simulink library "TrebleBoost"  (R2022b)
settings: Solver=VariableStepAuto  StartTime=0.0  StopTime=10.0  RelTol=1e-3
undefined symbols (not defined in the file or in its folder): magnitude, Row, TrebleBoost51Config, TrebleBoostConfig
libraries: TuneVar x30, TOP x12, StateVar x4, HandyTextFile x2, FeaturePath x2, PooliirLib x2, $bdroot x1, dspmtrx3 x1, dspxfrm3 x1
settings Model: Creator=jk1043656  LastModifiedBy=sc48041
settings SolverCC: AlgebraicLoopSolver=TrustRegion
settings DataIOCC: ReturnWorkspaceOutputs=off
settings DebuggingCC: UnconnectedInputMsg=warning  UnconnectedOutputMsg=warning  UnconnectedLineMsg=warning  SFMachineParentedDataDiag=warning  ArithmeticOperatorsInVariantConditions=warning
settings ModelReferenceCC: EnableRefExpFcnMdlSchedulingChecks=on
settings SFSimCC: CustomCodeUndefinedFunction=UseInterfaceOnly

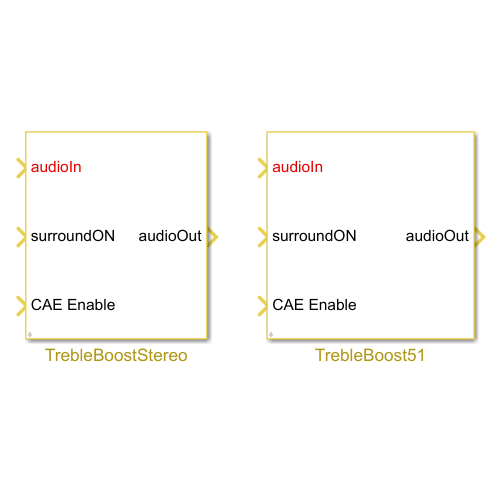
[thumbnail: Simulink's stored preview of the top-level diagram]
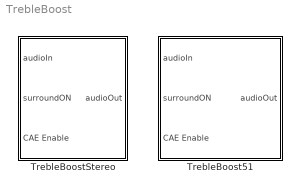
== system TrebleBoost ==
  TrebleBoost51 : Subsystem  mask{Config=TrebleBoost51Config}
      mask prompts: Config "TrebleBoost51Config"
      mask init:
      | blkh=gcbh;
      | Config=BTConfig.Assert(blkh,Config);
      | 
      | Config.Validate();
  TrebleBoostStereo : Subsystem  mask{Config=TrebleBoostConfig}
      mask prompts: Config "TrebleBoostStereoConfig"
      mask init:
      | blkh=gcbh;
      | Config=BTConfig.Assert(blkh,Config);
      | 
      | Config.Validate();

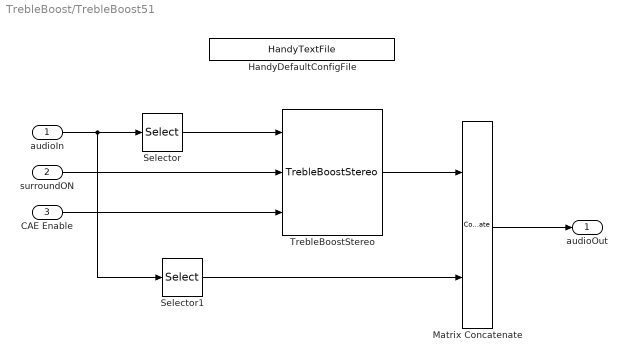
== system TrebleBoost/TrebleBoost51 ==
  audioIn : Inport  OutDataTypeStr=single
  surroundON : Inport  Port=2
  CAE Enable : Inport  Port=3
  HandyDefaultConfigFile : HandyTextFile/HandyTextFile  TemplateSource=Config  FileSuffix=Init  OpenDialogOnLoad=off  UseThisBlockName=off  AddGrandParentNamePrefix=off  TheDefaultText=|  ShowInLibBrowser=on
      | % $(FILENAME) Setup model parameters for each "Init" callback (e.g. update diagram)
      | sample_rate_in_hertz = 44100;
      | frame_size = 32;
      | sysin_channel_count = 2;
      settings: SourceProductName=Bose Talaria
  Matrix Concatenate : Concatenate  Mode=Multidimensional array  ConcatenateDimension=2
  Selector : Selector  NumberOfDimensions=2  InputPortWidth=3  IndexOptions=Select all,Index vector (dialog)  Indices=[1 3],[1 2]  OutputSizes=1,1
  Selector1 : Selector  NumberOfDimensions=2  InputPortWidth=3  IndexOptions=Select all,Index vector (dialog)  Indices=[1 3],3:6  OutputSizes=1,1
  TrebleBoostStereo : $bdroot/TrebleBoostStereo  Config=Config
  audioOut : Outport  OutDataTypeStr=single  VectorParamsAs1DForOutWhenUnconnected=off
  wires:
  Matrix Concatenate/1 -> audioOut/1
  Selector1/1 -> Matrix Concatenate/2
  audioIn/1 -> Selector/1, Selector1/1
  TrebleBoostStereo/1 -> Matrix Concatenate/1
  Selector/1 -> TrebleBoostStereo/1
  surroundON/1 -> TrebleBoostStereo/2
  CAE Enable/1 -> TrebleBoostStereo/3

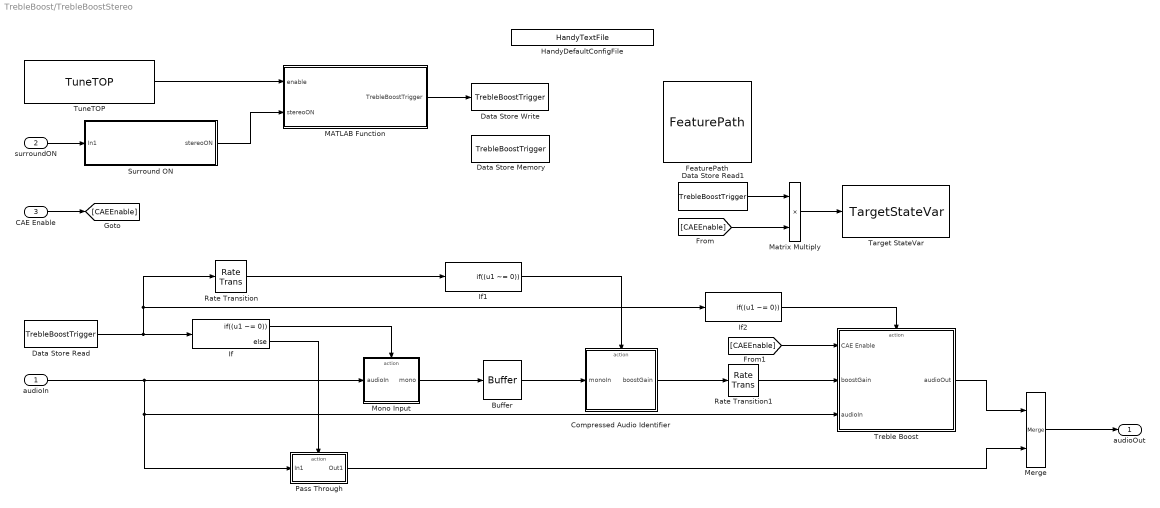
== system TrebleBoost/TrebleBoostStereo ==
  audioIn : Inport  OutDataTypeStr=single  PortDimensions=[32 2]
  surroundON : Inport  Port=2
  CAE Enable : Inport  Port=3
  Buffer : Buffer  N=Config.FftFrameSize  OutputFrames=off
  Compressed Audio Identifier : Subsystem  TreatAsAtomicUnit=on
  Data Store Memory : DataStoreMemory  DataStoreName=TrebleBoostTrigger  ReadBeforeWriteMsg=warning  WriteAfterWriteMsg=warning  WriteAfterReadMsg=warning  InitialValue=1  ShowAdditionalParam=off
  Data Store Read : DataStoreRead  DataStoreName=TrebleBoostTrigger  IndexOptions=Index vector (dialog)  Indices=1  OutputSizes=1
  Data Store Read1 : DataStoreRead  DataStoreName=TrebleBoostTrigger  IndexOptions=Index vector (dialog)  Indices=1  OutputSizes=1
  Data Store Write : DataStoreWrite  DataStoreName=TrebleBoostTrigger  IndexOptions=Index vector (dialog)  Indices=1  OutputSizes=1
  FeaturePath : FeaturePath/FeaturePath  FeatureName=TrebleBoost  IsGroup=off  GroupNumber=-1  IsModule=off  TriggerInit=[2025 269 2140 376]
      settings: SourceProductName=Bose Talaria
  HandyDefaultConfigFile : HandyTextFile/HandyTextFile  TemplateSource=Config  FileSuffix=Init  OpenDialogOnLoad=off  UseThisBlockName=off  AddGrandParentNamePrefix=off  TheDefaultText=|  ShowInLibBrowser=on
      | % $(FILENAME) Setup model parameters for each "Init" callback (e.g. update diagram)
      | sample_rate_in_hertz = 44100;
      | frame_size = 32;
      | sysin_channel_count = 2;
      settings: SourceProductName=Bose Talaria
  If : If  IfExpression=(u1 ~= 0)
  If1 : If  IfExpression=(u1 ~= 0)  ShowElse=off
  If2 : If  IfExpression=(u1 ~= 0)  ShowElse=off
  MATLAB Function : MATLAB Function  TreatAsAtomicUnit=on
  Matrix Multiply : Product  OutDataTypeStr=double
  Merge : Merge
  Mono Input : Subsystem  TreatAsAtomicUnit=on
  Pass Through : Subsystem  TreatAsAtomicUnit=on
  Rate Transition : RateTransition  Integrity=off  OutPortSampleTimeOpt=Multiple of input port sample time  OutPortSampleTimeMultiple=8
  Rate Transition1 : RateTransition  Integrity=off  OutPortSampleTimeOpt=Multiple of input port sample time  OutPortSampleTimeMultiple=1/8
  Surround ON : Subsystem
  Target StateVar : StateVar/TargetStateVar  TriggerInit=[2260 406 2400 474]  TspName=Enable  StateName=Enable  UseSameName=on  IfdefMacro=[]
      settings: SourceProductName=Bose Talaria
  Treble Boost : Subsystem  TreatAsAtomicUnit=on
  TuneTOP : TuneVar/TuneTOP  TriggerInit=[1190 242 1360 298]  TopName=EnableFlag  TuneName=EnableFlag  DataTypeOut=int32  TunabilityNumber=1  MinValue=[]  MaxValue=[]  BankNumber=0  PreOverlay=false  PostOverlay=false  UseSameName=on  MaskValue=Config.DefaultTuning.EnableFlag
      settings: SourceProductName=Bose Talaria
  audioOut : Outport  OutDataTypeStr=single  VectorParamsAs1DForOutWhenUnconnected=off
  wires:
  Rate Transition/1 -> If1/1
  If/2 -> Pass Through/Action
  MATLAB Function/1(TrebleBoostTrigger) -> Data Store Write/1
  Merge/1 -> audioOut/1
  Data Store Read/1 -> If/1, If2/1, Rate Transition/1
  Pass Through/1(Out1) -> Merge/2
  If2/1 -> Treble Boost/Action
  Treble Boost/1(audioOut) -> Merge/1
  Compressed Audio Identifier/1(boostGain) -> Rate Transition1/1
  Buffer/1 -> Compressed Audio Identifier/1(monoIn)
  Mono Input/1(mono) -> Buffer/1
  Rate Transition1/1 -> Treble Boost/2(boostGain)
  Surround ON/1(stereoON) -> MATLAB Function/2(stereoON)
  If/1 -> Mono Input/Action
  If1/1 -> Compressed Audio Identifier/Action
  surroundON/1 -> Surround ON/1(In1)
  audioIn/1 -> Pass Through/1(In1), Treble Boost/3(audioIn), Mono Input/1(audioIn)
  TuneTOP/1 -> MATLAB Function/1(enable)
  CAE Enable/1 -> [CAEEnable]
  [CAEEnable] -> Treble Boost/1(CAE Enable)
  Data Store Read1/1 -> Matrix Multiply/1
  [CAEEnable] -> Matrix Multiply/2
  Matrix Multiply/1 -> Target StateVar/1

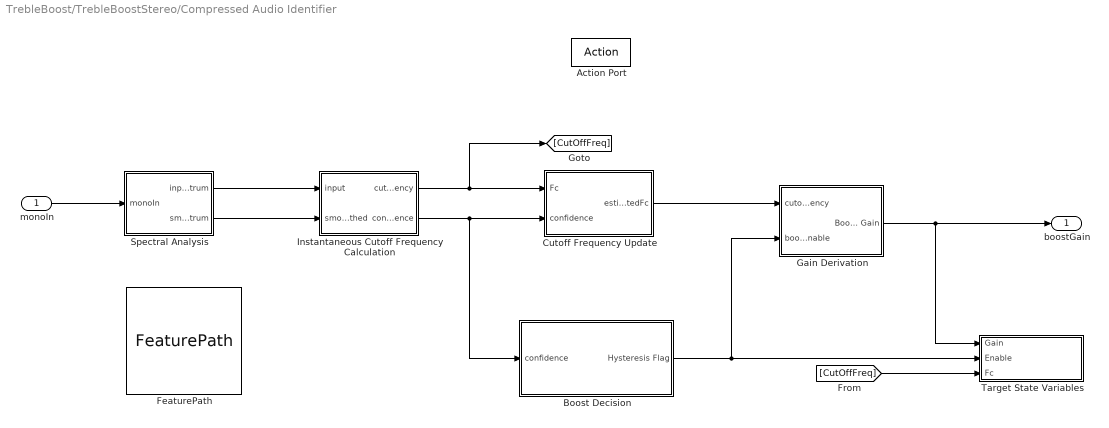
== system TrebleBoost/TrebleBoostStereo/Compressed Audio Identifier ==
  monoIn : Inport
  Action Port : ActionPort
  Boost Decision : Subsystem
  Cutoff Frequency Update : Subsystem
  FeaturePath : FeaturePath/FeaturePath  FeatureName=Identifier  IsGroup=off  GroupNumber=-1  IsModule=off  TriggerInit=[-155 264 -40 371]
      settings: SourceProductName=Bose Talaria
  Gain Derivation : Subsystem
  Instantaneous Cutoff Frequency Calculation : Subsystem
  Spectral Analysis : Subsystem
  Target State Variables : Subsystem
  boostGain : Outport  VectorParamsAs1DForOutWhenUnconnected=off
  wires:
  Gain Derivation/1(Boost Gain) -> boostGain/1, Target State Variables/1(Gain)
  Boost Decision/1(Hysteresis Flag) -> Gain Derivation/2(boostEnable), Target State Variables/2(Enable)
  Cutoff Frequency Update/1(estimatedFc) -> Gain Derivation/1(cutoffFrequency)
  Instantaneous Cutoff Frequency Calculation/1(cutoffFrequency) -> [CutOffFreq], Cutoff Frequency Update/1(Fc)
  monoIn/1 -> Spectral Analysis/1(monoIn)
  Instantaneous Cutoff Frequency Calculation/2(confidence) -> Boost Decision/1(confidence), Cutoff Frequency Update/2(confidence)
  Spectral Analysis/1(inputSpectrum) -> Instantaneous Cutoff Frequency Calculation/1(input)
  Spectral Analysis/2(smoothedSpectrum) -> Instantaneous Cutoff Frequency Calculation/2(smoothed)
  [CutOffFreq] -> Target State Variables/3(Fc)

== system TrebleBoost/TrebleBoostStereo/Mono Input ==
  audioIn : Inport
  Action Port : ActionPort
  Sum of Elements : Sum  Inputs=+  CollapseMode=Specified dimension  CollapseDim=2
  mono : Outport  VectorParamsAs1DForOutWhenUnconnected=off
  wires:
  audioIn/1 -> Sum of Elements/1
  Sum of Elements/1 -> mono/1

== system TrebleBoost/TrebleBoostStereo/Pass Through ==
  In1 : Inport
  Action Port : ActionPort
  Out1 : Outport  VectorParamsAs1DForOutWhenUnconnected=off
  wires:
  In1/1 -> Out1/1

== system TrebleBoost/TrebleBoostStereo/Surround ON ==
  In1 : Inport
  TOP : TOP/TOP  TriggerInit=[440 20 585 80]  TopName=StereoON  DataType=int32  BankNumber=0  PreOverlay=false  PostOverlay=false  Role=Automatic
      settings: SourceProductName=Bose Talaria
  TranslateTrigger : TuneVar/TranslateTrigger  TriggerInit=[306 -100 344 -45]
      settings: SourceProductName=Bose Talaria
  Trivial Translation : MATLAB Function  TreatAsAtomicUnit=on
  stereoON : Outport  VectorParamsAs1DForOutWhenUnconnected=off
  wires:
  TranslateTrigger/1 -> Trivial Translation/Trigger
  Trivial Translation/1(isStereo) -> TOP/1
  In1/1 -> Trivial Translation/1(surroundOn)  "SurroundON"
  TOP/1 -> stereoON/1  "StereoON"

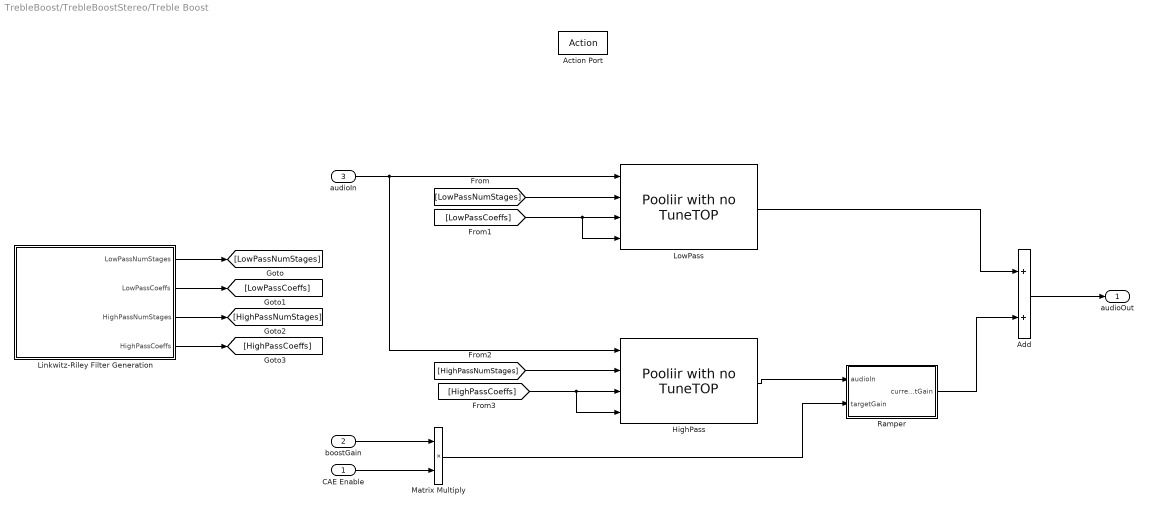
== system TrebleBoost/TrebleBoostStereo/Treble Boost ==
  CAE Enable : Inport
  boostGain : Inport  Port=2
  audioIn : Inport  Port=3
  Action Port : ActionPort
  Add : Sum
  HighPass : PooliirLib/Pooliir with no TuneTOP  maxNumStages=Config.MaxNumStages  variantType=Config.Variant
  Linkwitz-Riley Filter Generation : Subsystem
  LowPass : PooliirLib/Pooliir with no TuneTOP  maxNumStages=Config.MaxNumStages  variantType=Config.Variant
  Matrix Multiply : Product
  Ramper : Subsystem
  audioOut : Outport  VectorParamsAs1DForOutWhenUnconnected=off
  wires:
  Ramper/1(currentGain) -> Add/2
  HighPass/1 -> Ramper/1(audioIn)
  Linkwitz-Riley Filter Generation/3(HighPassNumStages) -> [HighPassNumStages]
  Linkwitz-Riley Filter Generation/1(LowPassNumStages) -> [LowPassNumStages]
  audioIn/1 -> LowPass/1, HighPass/1
  LowPass/1 -> Add/1
  [LowPassNumStages] -> LowPass/2
  [HighPassCoeffs] -> HighPass/4, HighPass/3
  Linkwitz-Riley Filter Generation/4(HighPassCoeffs) -> [HighPassCoeffs]
  [HighPassNumStages] -> HighPass/2
  Linkwitz-Riley Filter Generation/2(LowPassCoeffs) -> [LowPassCoeffs]
  [LowPassCoeffs] -> LowPass/4, LowPass/3
  Add/1 -> audioOut/1
  CAE Enable/1 -> Matrix Multiply/2
  boostGain/1 -> Matrix Multiply/1
  Matrix Multiply/1 -> Ramper/2(targetGain)

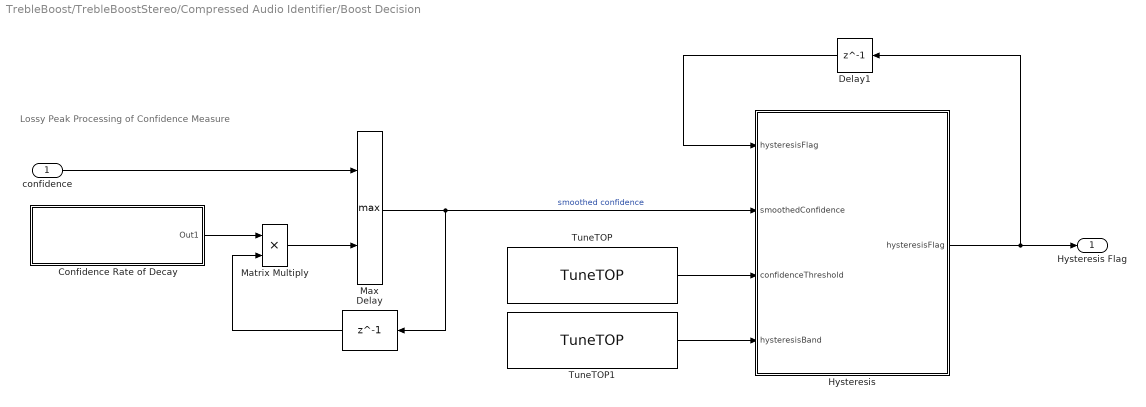
== system TrebleBoost/TrebleBoostStereo/Compressed Audio Identifier/Boost Decision ==
  note: Lossy Peak Processing of Confidence Measure
  confidence : Inport
  Confidence Rate of Decay : Subsystem
  Delay : Delay  DelayLength=1  InitialCondition=0
  Delay1 : Delay  DelayLength=1  InitialCondition=1
  Hysteresis : MATLAB Function  TreatAsAtomicUnit=on
  Matrix Multiply : Product
  Max : MinMax  Function=max  Inputs=2
  TuneTOP : TuneVar/TuneTOP  TriggerInit=[355 142 525 198]  TopName=ConfidenceThreshold  TuneName=ConfidenceThreshold  DataType=single  TunabilityNumber=1  MinValue=[]  MaxValue=[]  BankNumber=0  PreOverlay=false  PostOverlay=false  UseSameName=on  MaskValue=Config.DefaultTuning.ConfidenceThreshold
      settings: SourceProductName=Bose Talaria
  TuneTOP1 : TuneVar/TuneTOP  TriggerInit=[355 207 525 263]  TopName=HysteresisBand  TuneName=HysteresisBand  DataType=single  TunabilityNumber=1  MinValue=[]  MaxValue=[]  BankNumber=0  PreOverlay=false  PostOverlay=false  UseSameName=on  MaskValue=Config.DefaultTuning.HysteresisBand
      settings: SourceProductName=Bose Talaria
  Hysteresis Flag : Outport  VectorParamsAs1DForOutWhenUnconnected=off
  wires:
  Hysteresis/1(hysteresisFlag) -> Hysteresis Flag/1, Delay1/1
  TuneTOP1/1 -> Hysteresis/4(hysteresisBand)
  Matrix Multiply/1 -> Max/2
  Max/1 -> Delay/1, Hysteresis/2(smoothedConfidence)  "smoothed confidence"
  Confidence Rate of Decay/1(Out1) -> Matrix Multiply/1
  Delay/1 -> Matrix Multiply/2
  confidence/1 -> Max/1
  TuneTOP/1 -> Hysteresis/3(confidenceThreshold)
  Delay1/1 -> Hysteresis/1("hysteresisFlag ")

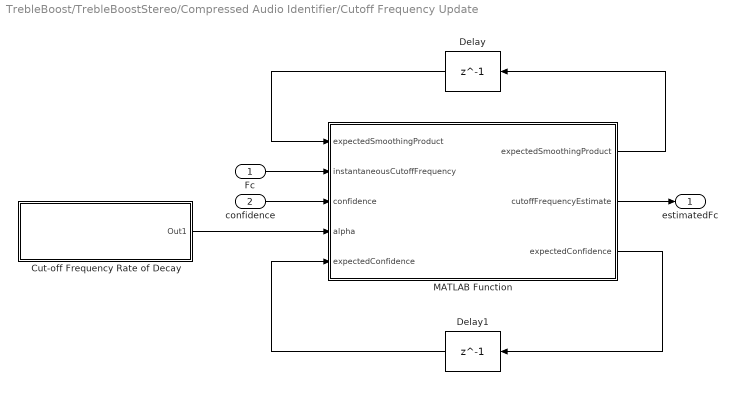
== system TrebleBoost/TrebleBoostStereo/Compressed Audio Identifier/Cutoff Frequency Update ==
  Fc : Inport
  confidence : Inport  Port=2
  Cut-off Frequency Rate of Decay : Subsystem
  Delay : Delay  DelayLength=1  InitialCondition=0
  Delay1 : Delay  DelayLength=1  InitialCondition=0
  MATLAB Function : MATLAB Function  TreatAsAtomicUnit=on
  estimatedFc : Outport  VectorParamsAs1DForOutWhenUnconnected=off
  wires:
  Cut-off Frequency Rate of Decay/1(Out1) -> MATLAB Function/4(alpha)
  confidence/1 -> MATLAB Function/3(confidence)
  Fc/1 -> MATLAB Function/2(instantaneousCutoffFrequency)
  MATLAB Function/3(expectedConfidence) -> Delay1/1
  Delay1/1 -> MATLAB Function/5("expectedConfidence ")
  Delay/1 -> MATLAB Function/1("expectedSmoothingProduct ")
  MATLAB Function/2(cutoffFrequencyEstimate) -> estimatedFc/1
  MATLAB Function/1(expectedSmoothingProduct) -> Delay/1

== system TrebleBoost/TrebleBoostStereo/Compressed Audio Identifier/Gain Derivation ==
  cutoffFrequency : Inport
  boostEnable : Inport  Port=2
  MATLAB Function : MATLAB Function  TreatAsAtomicUnit=on
  Subsystem : Subsystem
  Boost Gain : Outport  VectorParamsAs1DForOutWhenUnconnected=off
  wires:
  boostEnable/1 -> MATLAB Function/1(boostEnable)
  MATLAB Function/1(boostGain) -> Boost Gain/1
  Subsystem/1(Freq1InHz) -> MATLAB Function/3(Freq1Hz)
  Subsystem/2(Freq2InHz) -> MATLAB Function/4(Freq2Hz)
  Subsystem/3(Freq3InHz) -> MATLAB Function/5(Freq3Hz)
  Subsystem/4(Gain1IndB) -> MATLAB Function/6(Gain1dB)
  Subsystem/5(Gain2IndB) -> MATLAB Function/7(Gain2dB)
  cutoffFrequency/1 -> MATLAB Function/2(cutoffFrequency)

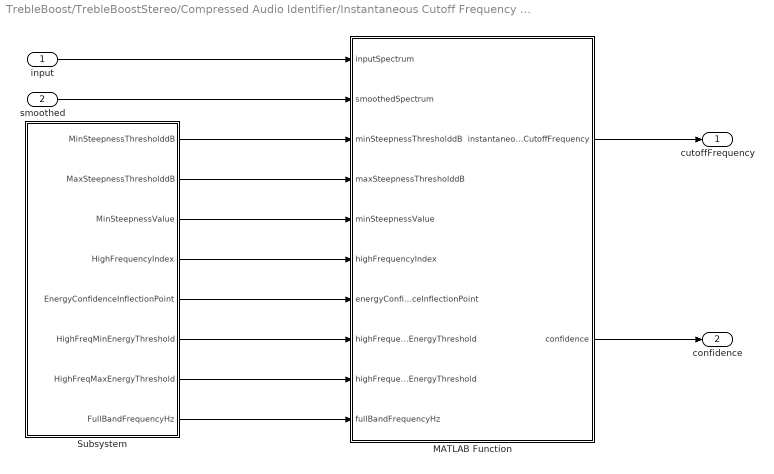
== system TrebleBoost/TrebleBoostStereo/Compressed Audio Identifier/Instantaneous Cutoff Frequency Calculation ==
  input : Inport
  smoothed : Inport  Port=2
  MATLAB Function : MATLAB Function  TreatAsAtomicUnit=on  mask{minDetectionFrequencyIndex=Config.MinDetectionFrequencyIndex, maxDetectionFrequencyIndex=Config.MaxDetectionFrequencyIndex, spectrumSize=Config.SpectrumSize, frequencies=Config.Frequencies, steepnessIndexRange=Config.SteepnessIndexRange}
  Subsystem : Subsystem
  cutoffFrequency : Outport  VectorParamsAs1DForOutWhenUnconnected=off
  confidence : Outport  Port=2  OutDataTypeStr=single  VectorParamsAs1DForOutWhenUnconnected=off
  wires:
  input/1 -> MATLAB Function/1(inputSpectrum)
  Subsystem/4(HighFrequencyIndex) -> MATLAB Function/6(highFrequencyIndex)
  Subsystem/8(FullBandFrequencyHz) -> MATLAB Function/10(fullBandFrequencyHz)
  Subsystem/7(HighFreqMaxEnergyThreshold) -> MATLAB Function/9(highFrequencyMaxEnergyThreshold)
  Subsystem/6(HighFreqMinEnergyThreshold) -> MATLAB Function/8(highFrequencyMinEnergyThreshold)
  Subsystem/5(EnergyConfidenceInflectionPoint) -> MATLAB Function/7(energyConfidenceInflectionPoint)
  Subsystem/3(MinSteepnessValue) -> MATLAB Function/5(minSteepnessValue)
  Subsystem/1(MinSteepnessThresholddB) -> MATLAB Function/3(minSteepnessThresholddB)
  MATLAB Function/2(confidence) -> confidence/1
  Subsystem/2(MaxSteepnessThresholddB) -> MATLAB Function/4(maxSteepnessThresholddB)
  MATLAB Function/1(instantaneousCutoffFrequency) -> cutoffFrequency/1
  smoothed/1 -> MATLAB Function/2(smoothedSpectrum)

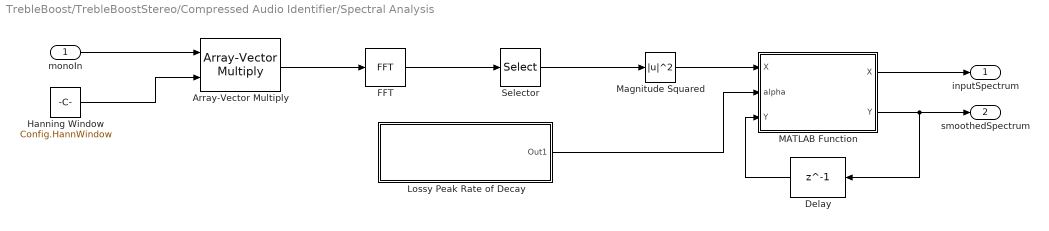
== system TrebleBoost/TrebleBoostStereo/Compressed Audio Identifier/Spectral Analysis ==
  monoIn : Inport
  Array-Vector Multiply : dspmtrx3/Array-Vector Multiply  mode=Mute  saveAsFlag=0  Dimension=1  V_Source=Input port  V_VectFromMask=[0.5 0.25]  roundingMode=Floor  overflowMode=off  firstCoeffSignedness=Auto  firstCoeffDataTypeStr=Inherit: Same word length as input  firstCoeffMin=[]  firstCoeffMax=[]  firstCoeffLastDataTypeStr=Inherit: Same word length as input  prodOutputSignedness=Auto  accumSignedness=Auto  outputSignedness=Auto  outputMin=[]  outputMax=[]
  Delay : Delay  DelayLength=1  InitialCondition=zeros(1, Config.SpectrumSize, 'single')
  FFT : dspxfrm3/FFT  FFTImplementation=Auto  CompMethod=Table lookup  TableOpt=NEW  TableOptActive=Speed  BitRevOrder=off  Normalize=off  InheritFFTLength=on  FFTLength=64  WrapInput=on  roundingMode=Floor  overflowMode=off  firstCoeffDataTypeStr=Inherit: Same word length as input  firstCoeffLastDataTypeStr=Inherit: Same word length as input  outputMin=[]  outputMax=[]
  Hanning Window : Constant  Value=Config.HannWindow  VectorParams1D=off  OutDataTypeStr=single  SampleTime=Inf
  Lossy Peak Rate of Decay : Subsystem
  MATLAB Function : MATLAB Function  TreatAsAtomicUnit=on  mask{spectrumSize=Config.SpectrumSize}
  Magnitude Squared : Math  Operator=magnitude^2  SignedPower=on
  Selector : Selector  NumberOfDimensions=2  InputPortWidth=3  IndexOptions=Index vector (dialog),Select all  Indices=1:Config.SpectrumSize,1  OutputSizes=1,1
  inputSpectrum : Outport  VectorParamsAs1DForOutWhenUnconnected=off
  smoothedSpectrum : Outport  Port=2  VectorParamsAs1DForOutWhenUnconnected=off
  wires:
  Array-Vector Multiply/1 -> FFT/1
  monoIn/1 -> Array-Vector Multiply/1
  FFT/1 -> Selector/1
  Hanning Window/1 -> Array-Vector Multiply/2
  Lossy Peak Rate of Decay/1(Out1) -> MATLAB Function/2(alpha)
  Magnitude Squared/1 -> MATLAB Function/1("X ")
  Selector/1 -> Magnitude Squared/1
  MATLAB Function/2(Y) -> smoothedSpectrum/1, Delay/1
  Delay/1 -> MATLAB Function/3("Y ")
  MATLAB Function/1(X) -> inputSpectrum/1

== system TrebleBoost/TrebleBoostStereo/Compressed Audio Identifier/Target State Variables ==
  Gain : Inport
  Enable : Inport  Port=2
  Fc : Inport  Port=3
  Target StateVar : StateVar/TargetStateVar  TriggerInit=[360 81 500 149]  TspName=BoostEnable  StateName=BoostEnable  UseSameName=on  IfdefMacro=[]
      settings: SourceProductName=Bose Talaria
  Target StateVar1 : StateVar/TargetStateVar  TriggerInit=[360 -4 500 64]  TspName=BoostGain  StateName=BoostGain  UseSameName=on  IfdefMacro=[]
      settings: SourceProductName=Bose Talaria
  Target StateVar2 : StateVar/TargetStateVar  TriggerInit=[360 166 500 234]  TspName=CutOffFrequency  StateName=CutOffFrequency  UseSameName=on  IfdefMacro=[]
      settings: SourceProductName=Bose Talaria
  wires:
  Fc/1 -> Target StateVar2/1
  Gain/1 -> Target StateVar1/1
  Enable/1 -> Target StateVar/1

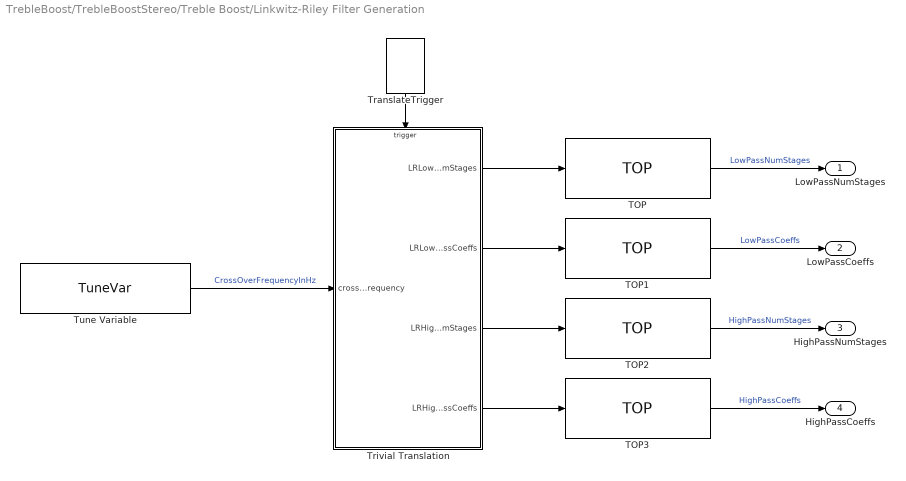
== system TrebleBoost/TrebleBoostStereo/Treble Boost/Linkwitz-Riley Filter Generation ==
  TOP : TOP/TOP  TriggerInit=[490 -25 635 35]  TopName=LowPassNumStages  DataType=uint32  BankNumber=0  PreOverlay=false  PostOverlay=false  Role=Automatic
      settings: SourceProductName=Bose Talaria
  TOP1 : TOP/TOP  TriggerInit=[490 55 635 115]  TopName=LowPassCoeffs  DataType=single  BankNumber=0  PreOverlay=false  PostOverlay=false  Role=Automatic
      settings: SourceProductName=Bose Talaria
  TOP2 : TOP/TOP  TriggerInit=[490 135 635 195]  TopName=HighPassNumStages  DataType=uint32  BankNumber=0  PreOverlay=false  PostOverlay=false  Role=Automatic
      settings: SourceProductName=Bose Talaria
  TOP3 : TOP/TOP  TriggerInit=[490 215 635 275]  TopName=HighPassCoeffs  DataType=single  BankNumber=0  PreOverlay=false  PostOverlay=false  Role=Automatic
      settings: SourceProductName=Bose Talaria
  TranslateTrigger : TuneVar/TranslateTrigger  TriggerInit=[311 -125 349 -70]
      settings: SourceProductName=Bose Talaria
  Trivial Translation : MATLAB Function  TreatAsAtomicUnit=on  mask{filterOrder=Config.FilterOrder, sampleRate=Config.SampleRate, maxNumStages=Config.MaxNumStages, numChannels=Config.NumChannels}
  Tune Variable : TuneVar/TuneVar  TuneName=CrossOverFrequencyInHz  SpecifyMaxSize=off  VariableDim=1 (Row)  MaxSize=[1 1]  TunabilityNumber=1  MinValue=[]  MaxValue=[]  TriggerInit=[-55 100 115 150]  MaskValue=Config.DefaultTuning.CrossOverFrequency
      settings: SourceProductName=Bose Talaria
  LowPassNumStages : Outport  VectorParamsAs1DForOutWhenUnconnected=off
  LowPassCoeffs : Outport  Port=2  VectorParamsAs1DForOutWhenUnconnected=off
  HighPassNumStages : Outport  Port=3  VectorParamsAs1DForOutWhenUnconnected=off
  HighPassCoeffs : Outport  Port=4  VectorParamsAs1DForOutWhenUnconnected=off
  wires:
  Trivial Translation/4(LRHighPassCoeffs) -> TOP3/1
  Trivial Translation/3(LRHighPassNumStages) -> TOP2/1
  Trivial Translation/2(LRLowPassCoeffs) -> TOP1/1
  TOP3/1 -> HighPassCoeffs/1  "HighPassCoeffs"
  TOP2/1 -> HighPassNumStages/1  "HighPassNumStages"
  TOP1/1 -> LowPassCoeffs/1  "LowPassCoeffs"
  TranslateTrigger/1 -> Trivial Translation/Trigger
  Trivial Translation/1(LRLowPassNumStages) -> TOP/1
  Tune Variable/1 -> Trivial Translation/1(crossOverFrequency)  "CrossOverFrequencyInHz"
  TOP/1 -> LowPassNumStages/1  "LowPassNumStages"

== system TrebleBoost/TrebleBoostStereo/Treble Boost/Ramper ==
  audioIn : Inport
  targetGain : Inport  Port=2
  MATLAB Function : MATLAB Function  TreatAsAtomicUnit=on
  Ramp Coefficient : Subsystem
  currentGain : Outport  VectorParamsAs1DForOutWhenUnconnected=off
  wires:
  MATLAB Function/1(audioOut) -> currentGain/1
  targetGain/1 -> MATLAB Function/2(targetGain)
  audioIn/1 -> MATLAB Function/1(audioIn)
  Ramp Coefficient/1(RampCoef) -> MATLAB Function/3(rampCoef)

== system TrebleBoost/TrebleBoostStereo/Compressed Audio Identifier/Boost Decision/Confidence Rate of Decay ==
  TOP : TOP/TOP  TriggerInit=[470 20 615 80]  TopName=ConfidenceAlpha  DataType=single  BankNumber=0  PreOverlay=false  PostOverlay=false  Role=Automatic
      settings: SourceProductName=Bose Talaria
  TranslateTrigger : TuneVar/TranslateTrigger  TriggerInit=[306 -100 344 -45]
      settings: SourceProductName=Bose Talaria
  Trivial Translation : MATLAB Function  TreatAsAtomicUnit=on  mask{sampleRate=Config.SampleRate, fftFrameSize=Config.FftFrameSize}
  Tune Variable : TuneVar/TuneVar  TuneName=ConfidenceTau  SpecifyMaxSize=on  VariableDim=1 (Row)  MaxSize=[1 1]  TunabilityNumber=1  MinValue=[]  MaxValue=[]  TriggerInit=[-60 25 165 75]  MaskValue=Config.DefaultTuning.ConfidenceTau
      settings: SourceProductName=Bose Talaria
  Out1 : Outport  VectorParamsAs1DForOutWhenUnconnected=off
  wires:
  TranslateTrigger/1 -> Trivial Translation/Trigger
  Trivial Translation/1(decay) -> TOP/1
  Tune Variable/1 -> Trivial Translation/1(timeConstant)  "ConfidenceTau"
  TOP/1 -> Out1/1  "ConfidenceAlpha"

== system TrebleBoost/TrebleBoostStereo/Compressed Audio Identifier/Cutoff Frequency Update/Cut-off Frequency Rate of Decay ==
  TOP : TOP/TOP  TriggerInit=[470 20 615 80]  TopName=CutoffFrequencyAlpha  DataType=single  BankNumber=0  PreOverlay=false  PostOverlay=false  Role=Automatic
      settings: SourceProductName=Bose Talaria
  TranslateTrigger : TuneVar/TranslateTrigger  TriggerInit=[306 -100 344 -45]
      settings: SourceProductName=Bose Talaria
  Trivial Translation : MATLAB Function  TreatAsAtomicUnit=on  mask{sampleRate=Config.SampleRate, fftFrameSize=Config.FftFrameSize}
  Tune Variable : TuneVar/TuneVar  TuneName=CutoffFrequencyTau  SpecifyMaxSize=on  VariableDim=1 (Row)  MaxSize=[1 1]  TunabilityNumber=1  MinValue=[]  MaxValue=[]  TriggerInit=[-60 25 165 75]  MaskValue=Config.DefaultTuning.CutoffFrequencyTau
      settings: SourceProductName=Bose Talaria
  Out1 : Outport  VectorParamsAs1DForOutWhenUnconnected=off
  wires:
  TranslateTrigger/1 -> Trivial Translation/Trigger
  Trivial Translation/1(decay) -> TOP/1
  Tune Variable/1 -> Trivial Translation/1(timeConstant)  "CutoffFrequencyTau"
  TOP/1 -> Out1/1  "CutoffFrequencyAlpha"

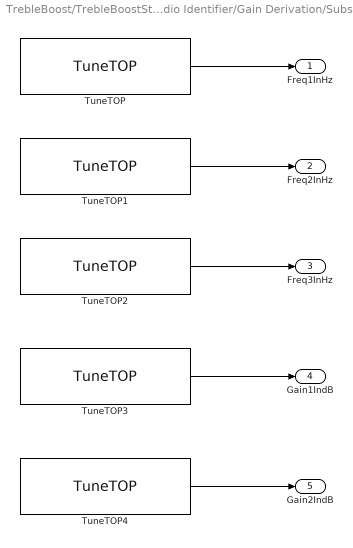
== system TrebleBoost/TrebleBoostStereo/Compressed Audio Identifier/Gain Derivation/Subsystem ==
  TuneTOP : TuneVar/TuneTOP  TriggerInit=[-95 -143 75 -87]  TopName=Freq1InHz  TuneName=Freq1InHz  DataType=single  TunabilityNumber=2  MinValue=[]  MaxValue=[]  BankNumber=0  PreOverlay=false  PostOverlay=false  UseSameName=on  MaskValue=Config.DefaultTuning.Freq1InHz
      settings: SourceProductName=Bose Talaria
  TuneTOP1 : TuneVar/TuneTOP  TriggerInit=[-95 -43 75 13]  TopName=Freq2InHz  TuneName=Freq2InHz  DataType=single  TunabilityNumber=2  MinValue=[]  MaxValue=[]  BankNumber=0  PreOverlay=false  PostOverlay=false  UseSameName=on  MaskValue=Config.DefaultTuning.Freq2InHz
      settings: SourceProductName=Bose Talaria
  TuneTOP2 : TuneVar/TuneTOP  TriggerInit=[-95 57 75 113]  TopName=Freq3InHz  TuneName=Freq3InHz  DataType=single  TunabilityNumber=2  MinValue=[]  MaxValue=[]  BankNumber=0  PreOverlay=false  PostOverlay=false  UseSameName=on  MaskValue=Config.DefaultTuning.Freq3InHz
      settings: SourceProductName=Bose Talaria
  TuneTOP3 : TuneVar/TuneTOP  TriggerInit=[-95 167 75 223]  TopName=Gain1IndB  TuneName=Gain1IndB  DataType=single  TunabilityNumber=1  MinValue=[]  MaxValue=[]  BankNumber=0  PreOverlay=false  PostOverlay=false  UseSameName=on  MaskValue=Config.DefaultTuning.Gain1IndB
      settings: SourceProductName=Bose Talaria
  TuneTOP4 : TuneVar/TuneTOP  TriggerInit=[-95 277 75 333]  TopName=Gain2IndB  TuneName=Gain2IndB  DataType=single  TunabilityNumber=1  MinValue=[]  MaxValue=[]  BankNumber=0  PreOverlay=false  PostOverlay=false  UseSameName=on  MaskValue=Config.DefaultTuning.Gain2IndB
      settings: SourceProductName=Bose Talaria
  Freq1InHz : Outport
  Freq2InHz : Outport  Port=2
  Freq3InHz : Outport  Port=3
  Gain1IndB : Outport  Port=4
  Gain2IndB : Outport  Port=5
  wires:
  TuneTOP/1 -> Freq1InHz/1
  TuneTOP1/1 -> Freq2InHz/1
  TuneTOP2/1 -> Freq3InHz/1
  TuneTOP3/1 -> Gain1IndB/1
  TuneTOP4/1 -> Gain2IndB/1

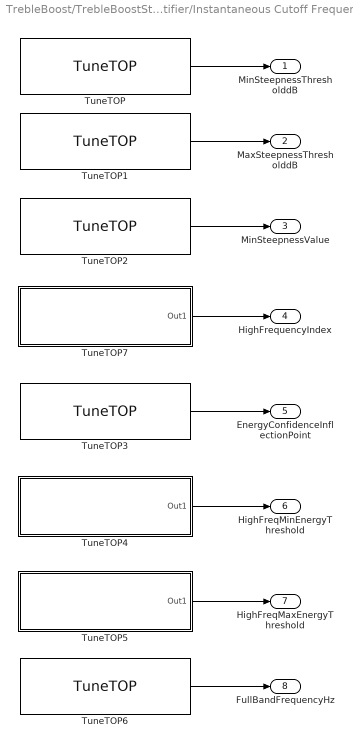
== system TrebleBoost/TrebleBoostStereo/Compressed Audio Identifier/Instantaneous Cutoff Frequency Calculation/Subsystem ==
  TuneTOP : TuneVar/TuneTOP  TriggerInit=[20 17 190 73]  TopName=MinSteepnessThresholddB  TuneName=MinSteepnessThresholddB  DataType=single  TunabilityNumber=1  MinValue=[]  MaxValue=[]  BankNumber=0  PreOverlay=false  PostOverlay=false  UseSameName=on  MaskValue=Config.DefaultTuning.MinSteepnessThresholddB
      settings: SourceProductName=Bose Talaria
  TuneTOP1 : TuneVar/TuneTOP  TriggerInit=[20 92 190 148]  TopName=MaxSteepnessThresholddB  TuneName=MaxSteepnessThresholddB  DataType=single  TunabilityNumber=1  MinValue=[]  MaxValue=[]  BankNumber=0  PreOverlay=false  PostOverlay=false  UseSameName=on  MaskValue=Config.DefaultTuning.MaxSteepnessThresholddB
      settings: SourceProductName=Bose Talaria
  TuneTOP2 : TuneVar/TuneTOP  TriggerInit=[20 177 190 233]  TopName=MinSteepnessValue  TuneName=MinSteepnessValue  DataType=single  TunabilityNumber=1  MinValue=[]  MaxValue=[]  BankNumber=0  PreOverlay=false  PostOverlay=false  UseSameName=on  MaskValue=Config.DefaultTuning.MinSteepnessValue
      settings: SourceProductName=Bose Talaria
  TuneTOP3 : TuneVar/TuneTOP  TriggerInit=[20 362 190 418]  TopName=EnergyConfidenceInflectionPoint  TuneName=EnergyConfidenceInflectionPoint  DataType=single  TunabilityNumber=1  MinValue=[]  MaxValue=[]  BankNumber=0  PreOverlay=false  PostOverlay=false  UseSameName=on  MaskValue=Config.DefaultTuning.EnergyConfidenceInflectionPoint
      settings: SourceProductName=Bose Talaria
  TuneTOP4 : Subsystem
  TuneTOP5 : Subsystem
  TuneTOP6 : TuneVar/TuneTOP  TriggerInit=[20 637 190 693]  TopName=FullBandFrequencyHz  TuneName=FullBandFrequencyHz  DataType=single  TunabilityNumber=1  MinValue=[]  MaxValue=[]  BankNumber=0  PreOverlay=false  PostOverlay=false  UseSameName=on  MaskValue=Config.DefaultTuning.FullBandFrequencyHz
      settings: SourceProductName=Bose Talaria
  TuneTOP7 : Subsystem
  MinSteepnessThresholddB : Outport  VectorParamsAs1DForOutWhenUnconnected=off
  MaxSteepnessThresholddB : Outport  Port=2  VectorParamsAs1DForOutWhenUnconnected=off
  MinSteepnessValue : Outport  Port=3  VectorParamsAs1DForOutWhenUnconnected=off
  HighFrequencyIndex : Outport  Port=4  VectorParamsAs1DForOutWhenUnconnected=off
  EnergyConfidenceInflectionPoint : Outport  Port=5  VectorParamsAs1DForOutWhenUnconnected=off
  HighFreqMinEnergyThreshold : Outport  Port=6  VectorParamsAs1DForOutWhenUnconnected=off
  HighFreqMaxEnergyThreshold : Outport  Port=7  VectorParamsAs1DForOutWhenUnconnected=off
  FullBandFrequencyHz : Outport  Port=8  VectorParamsAs1DForOutWhenUnconnected=off
  wires:
  TuneTOP7/1(Out1) -> HighFrequencyIndex/1
  TuneTOP6/1 -> FullBandFrequencyHz/1
  TuneTOP5/1(Out1) -> HighFreqMaxEnergyThreshold/1
  TuneTOP4/1(Out1) -> HighFreqMinEnergyThreshold/1
  TuneTOP3/1 -> EnergyConfidenceInflectionPoint/1
  TuneTOP/1 -> MinSteepnessThresholddB/1
  TuneTOP2/1 -> MinSteepnessValue/1
  TuneTOP1/1 -> MaxSteepnessThresholddB/1

== system TrebleBoost/TrebleBoostStereo/Compressed Audio Identifier/Spectral Analysis/Lossy Peak Rate of Decay ==
  TOP : TOP/TOP  TriggerInit=[440 20 585 80]  TopName=LossyPeakAlpha  DataType=single  BankNumber=0  PreOverlay=false  PostOverlay=false  Role=Automatic
      settings: SourceProductName=Bose Talaria
  TranslateTrigger : TuneVar/TranslateTrigger  TriggerInit=[306 -100 344 -45]
      settings: SourceProductName=Bose Talaria
  Trivial Translation : MATLAB Function  TreatAsAtomicUnit=on  mask{sampleRate=Config.SampleRate, fftFrameSize=Config.FftFrameSize}
  Tune Variable : TuneVar/TuneVar  TuneName=LossyPeakTau  SpecifyMaxSize=on  VariableDim=1 (Row)  MaxSize=[1 1]  TunabilityNumber=1  MinValue=[]  MaxValue=[]  TriggerInit=[-5 25 195 75]  MaskValue=Config.DefaultTuning.LossyPeakTau
      settings: SourceProductName=Bose Talaria
  Out1 : Outport  VectorParamsAs1DForOutWhenUnconnected=off
  wires:
  TranslateTrigger/1 -> Trivial Translation/Trigger
  Trivial Translation/1(decay) -> TOP/1
  Tune Variable/1 -> Trivial Translation/1(timeConstant)  "LossyPeakTau"
  TOP/1 -> Out1/1  "LossyPeakAlpha"

== system TrebleBoost/TrebleBoostStereo/Treble Boost/Ramper/Ramp Coefficient ==
  TOP : TOP/TOP  TriggerInit=[470 20 615 80]  TopName=RampCoef  DataType=single  BankNumber=0  PreOverlay=false  PostOverlay=false  Role=Automatic
      settings: SourceProductName=Bose Talaria
  TranslateTrigger : TuneVar/TranslateTrigger  TriggerInit=[306 -100 344 -45]
      settings: SourceProductName=Bose Talaria
  Trivial Translation : MATLAB Function  TreatAsAtomicUnit=on  mask{sampleRate=Config.SampleRate}
  Tune Variable : TuneVar/TuneVar  TuneName=RamperTau  SpecifyMaxSize=on  VariableDim=1 (Row)  MaxSize=[1 1]  TunabilityNumber=1  MinValue=[]  MaxValue=[]  TriggerInit=[-60 25 165 75]  MaskValue=Config.DefaultTuning.RamperTau
      settings: SourceProductName=Bose Talaria
  RampCoef : Outport  VectorParamsAs1DForOutWhenUnconnected=off
  wires:
  TOP/1 -> RampCoef/1  "RampCoef"
  Tune Variable/1 -> Trivial Translation/1(timeConstant)  "RamperTau"
  Trivial Translation/1(rampCoef) -> TOP/1
  TranslateTrigger/1 -> Trivial Translation/Trigger

== system TrebleBoost/TrebleBoostStereo/Compressed Audio Identifier/Instantaneous Cutoff Frequency Calculation/Subsystem/TuneTOP4 ==
  TOP : TOP/TOP  TriggerInit=[440 20 585 80]  TopName=HighFrequencyMinEnergyThreshold  DataType=single  BankNumber=0  PreOverlay=false  PostOverlay=false  Role=Automatic
      settings: SourceProductName=Bose Talaria
  TranslateTrigger : TuneVar/TranslateTrigger  TriggerInit=[311 -100 349 -45]
      settings: SourceProductName=Bose Talaria
  Trivial Translation : MATLAB Function  TreatAsAtomicUnit=on
  Tune Variable : TuneVar/TuneVar  TuneName=HighFrequencyMinEnergyThresholddB  SpecifyMaxSize=off  VariableDim=1 (Row)  MaxSize=[1 1]  TunabilityNumber=1  MinValue=[]  MaxValue=[]  TriggerInit=[-85 25 85 75]  MaskValue=Config.DefaultTuning.HighFrequencyMinEnergyThresholddB
      settings: SourceProductName=Bose Talaria
  Out1 : Outport  VectorParamsAs1DForOutWhenUnconnected=off
  wires:
  TranslateTrigger/1 -> Trivial Translation/Trigger
  Trivial Translation/1(threshold_linear) -> TOP/1
  Tune Variable/1 -> Trivial Translation/1(threshold_dB)  "HighFrequencyMinEnergyThresholddB"
  TOP/1 -> Out1/1  "HighFrequencyMinEnergyThreshold"

== system TrebleBoost/TrebleBoostStereo/Compressed Audio Identifier/Instantaneous Cutoff Frequency Calculation/Subsystem/TuneTOP5 ==
  TOP : TOP/TOP  TriggerInit=[440 20 585 80]  TopName=HighFrequencyMaxEnergyThreshold  DataType=single  BankNumber=0  PreOverlay=false  PostOverlay=false  Role=Automatic
      settings: SourceProductName=Bose Talaria
  TranslateTrigger : TuneVar/TranslateTrigger  TriggerInit=[311 -100 349 -45]
      settings: SourceProductName=Bose Talaria
  Trivial Translation : MATLAB Function  TreatAsAtomicUnit=on
  Tune Variable : TuneVar/TuneVar  TuneName=HighFrequencyMaxEnergyThresholddB  SpecifyMaxSize=off  VariableDim=1 (Row)  MaxSize=[1 1]  TunabilityNumber=1  MinValue=[]  MaxValue=[]  TriggerInit=[-90 25 80 75]  MaskValue=Config.DefaultTuning.HighFrequencyMaxEnergyThresholddB
      settings: SourceProductName=Bose Talaria
  Out1 : Outport  VectorParamsAs1DForOutWhenUnconnected=off
  wires:
  TranslateTrigger/1 -> Trivial Translation/Trigger
  Trivial Translation/1(threshold_linear) -> TOP/1
  Tune Variable/1 -> Trivial Translation/1(threshold_dB)  "HighFrequencyMaxEnergyThresholddB"
  TOP/1 -> Out1/1  "HighFrequencyMaxEnergyThreshold"

== system TrebleBoost/TrebleBoostStereo/Compressed Audio Identifier/Instantaneous Cutoff Frequency Calculation/Subsystem/TuneTOP7 ==
  TOP : TOP/TOP  TriggerInit=[440 20 585 80]  TopName=HighFrequencyIndex  DataType=int32  BankNumber=0  PreOverlay=false  PostOverlay=false  Role=Automatic
      settings: SourceProductName=Bose Talaria
  TranslateTrigger : TuneVar/TranslateTrigger  TriggerInit=[306 -100 344 -45]
      settings: SourceProductName=Bose Talaria
  Trivial Translation : MATLAB Function  TreatAsAtomicUnit=on  mask{sampleRate=Config.SampleRate, fftFrameSize=Config.FftFrameSize}
  Tune Variable : TuneVar/TuneVar  TuneName=HighFrequency  SpecifyMaxSize=off  VariableDim=1 (Row)  MaxSize=[1 1]  TunabilityNumber=1  MinValue=[]  MaxValue=[]  TriggerInit=[20 25 190 75]  MaskValue=Config.DefaultTuning.HighFrequency
      settings: SourceProductName=Bose Talaria
  Out1 : Outport  VectorParamsAs1DForOutWhenUnconnected=off
  wires:
  TranslateTrigger/1 -> Trivial Translation/Trigger
  Trivial Translation/1(index) -> TOP/1
  Tune Variable/1 -> Trivial Translation/1(highFrequency)  "HighFrequency"
  TOP/1 -> Out1/1  "HighFrequencyIndex"

== matlab function TrebleBoost/TrebleBoostStereo/Compressed Audio Identifier/Instantaneous Cutoff Frequency Calculation/Subsystem/TuneTOP4/Trivial Translation ==
  data: threshold_linear output; threshold_dB input
  events: trigger input FUNCTION_CALL_EVENT
function threshold_linear  = fcn(threshold_dB)
%#codegen

threshold_dB = threshold_dB.Value;

threshold_linear = 10^(threshold_dB/10);

end

== matlab function TrebleBoost/TrebleBoostStereo/Compressed Audio Identifier/Instantaneous Cutoff Frequency Calculation/Subsystem/TuneTOP5/Trivial Translation ==
  data: threshold_linear output; threshold_dB input
  events: trigger input FUNCTION_CALL_EVENT
function threshold_linear  = fcn(threshold_dB)
%#codegen

threshold_dB = threshold_dB.Value;

threshold_linear = 10^(threshold_dB/10);

end

== matlab function TrebleBoost/TrebleBoostStereo/Compressed Audio Identifier/Instantaneous Cutoff Frequency Calculation/Subsystem/TuneTOP7/Trivial Translation ==
  data: index output; highFrequency input; sampleRate parameter; fftFrameSize parameter
  events: trigger input FUNCTION_CALL_EVENT
function index  = fcn(highFrequency, sampleRate, fftFrameSize)
%#codegen
%[Param:sampleRate]
%[Param:fftFrameSize]

highFreq = highFrequency.Value;

index = floor((highFreq/(sampleRate/2)) * (fftFrameSize/2));

end

== matlab function TrebleBoost/TrebleBoostStereo/Compressed Audio Identifier/Spectral Analysis/Lossy Peak Rate of Decay/Trivial Translation ==
  data: decay output; timeConstant input; sampleRate parameter; fftFrameSize parameter
  events: trigger input FUNCTION_CALL_EVENT
function decay  = fcn(timeConstant, sampleRate, fftFrameSize)
%#codegen
%[Param:sampleRate]
%[Param:fftFrameSize]
tau = timeConstant.Value;
Fd = sampleRate/fftFrameSize;
wc = 1/(tau*Fd);

decay = 1 - ((1-sin(wc))/cos(wc));

end

== matlab function TrebleBoost/TrebleBoostStereo/Compressed Audio Identifier/Spectral Analysis/MATLAB Function ==
  data: X output; X input single; alpha input; Y input single; Y output; spectrumSize parameter
function [X,Y] = LossyPeak(X,alpha, Y, spectrumSize)
% #codegen
%[Param:spectrumSize]

% % The Nyquist value is set to 0, because currently the Sharc library
% % functions, rfftN(), do not return the Nyquist values.  We will,
% % however, proceed as if that value is there but merely zero.
% X(Config.spectrumSize) = 0;

for i = 1:spectrumSize
    if (X(i) > Y(i))
        Y(i) = X(i);
    else
        Y(i)= ((1-alpha)*Y(i) + alpha*X(i));
    end
end

end

== matlab function TrebleBoost/TrebleBoostStereo/MATLAB Function ==
  data: enable input; stereoON input; TrebleBoostTrigger output
function TrebleBoostTrigger = trigger(enable, stereoON)
%#codegen
TrebleBoostTrigger = enable*stereoON;

== matlab function TrebleBoost/TrebleBoostStereo/Surround ON/Trivial Translation ==
  data: isStereo output; surroundOn input
  events: trigger input FUNCTION_CALL_EVENT
function isStereo  = checkStereo(surroundOn)
%#codegen

if(surroundOn.Value == 0 || surroundOn.Value == 2)
    isStereo = true;
else
    isStereo = false;
end

== matlab function TrebleBoost/TrebleBoostStereo/Treble Boost/Linkwitz-Riley Filter Generation/Trivial Translation ==
  data: crossOverFrequency input; LRLowPassNumStages output; LRLowPassCoeffs output; LRHighPassNumStages output; LRHighPassCoeffs output; filterOrder parameter; sampleRate parameter; maxNumStages parameter; numChannels parameter
  events: trigger input FUNCTION_CALL_EVENT
function [LRLowPassNumStages, LRLowPassCoeffs, LRHighPassNumStages, LRHighPassCoeffs]  = fcn(crossOverFrequency, filterOrder, sampleRate, maxNumStages, numChannels)
%#codegen
%[Param:filterOrder]
%[Param:sampleRate]
%[Param:maxNumStages]
%[Param:numChannels]

% Linkwitz-Riley Filters can be construed as the cascade of
% two Butterworth Filters of half the order at the same frequency.

butterOrder = filterOrder/2;
normFrequency = crossOverFrequency.Value/(sampleRate/2);

% Low-pass Filters
[halfZ, halfP, halfK] = butter_for_code_gen(butterOrder,butterOrder,normFrequency,'low');
fullZ = [halfZ halfZ];                         % zeros
fullP = [halfP halfP];                         % poles
fullK = halfK*halfK;                           % gain
sosLowPass = zp2sos_for_code_gen(fullZ,fullP,fullK);

% High-pass Filters
[halfZ, halfP, halfK] = butter_for_code_gen(butterOrder,butterOrder,normFrequency,'high');
fullZ = [halfZ halfZ];                         % zeros
fullP = [halfP halfP];                         % poles
fullK = halfK*halfK;                           % gain
sosHighPass = zp2sos_for_code_gen(fullZ,fullP,fullK);

% Generate Linkwitz-Riley Pair Coefficients
numStages = size(sosLowPass, 1) * ones(1, numChannels);
rawSOSLowPass = repmat(sosLowPass, numChannels, 1);
[LRLowPassNumStages, LRLowPassCoeffs] = pooliirTranslation(rawSOSLowPass, numStages, maxNumStages);

numStages = size(sosHighPass, 1) * ones(1, numChannels);
rawSOSHighPass = repmat(sosHighPass, numChannels, 1);
[LRHighPassNumStages, LRHighPassCoeffs] = pooliirTranslation(rawSOSHighPass, numStages, maxNumStages);

end

function [PoolNumStages, PoolCoeffs] = pooliirTranslation(rawSOS, numStages, maxNumStages)

RawSOS = rawSOS;
NumStages = int32(numStages);
NumChannels = length(NumStages);

MaxNumStages = maxNumStages; 
PoolNumStages = int32(zeros(NumChannels,1));
PoolCoeffs = single(zeros(MaxNumStages * 4 + NumChannels,1));
ChannelCoeffs = zeros(MaxNumStages * 4 + 1,1);
ChannelSOS = single(zeros(MaxNumStages, 6));
SOSIndex = int32(0);


for i = 1:NumChannels
    
    ChannelNumStages = NumStages(i);   % Size of current SOS
    assert(ChannelNumStages <= MaxNumStages);
    
    if (ChannelNumStages == 0)
        continue;
    end
    
    ChannelSOS(1:ChannelNumStages,:) = RawSOS(SOSIndex+(1:ChannelNumStages),:);
    SOSIndex = SOSIndex + ChannelNumStages;

    if size(ChannelSOS,2) ~= 6
        TranslateError('SOS matrix must have 6 columns');
    end
    % decompose SOS
   
    ts = 1:4:4*ChannelNumStages;
    ChannelCoeffs(1,1) = prod(ChannelSOS(1:ChannelNumStages,1));        % b0
	
	% Error out for poorly-formed sos coeffs
	if ((ChannelCoeffs(1,1) == 0) && (ChannelNumStages > 1))
		TranslateError('Poorly-formed SOS: zero b0 for multi-stage results in a zero EQ.');
	end
    
    % the remaining coeffs are compacted forms of the biquads
    ChannelCoeffs(1+ts,1) = ChannelSOS(1:ChannelNumStages,6);           % a2
    ChannelCoeffs(2+ts,1) = ChannelSOS(1:ChannelNumStages,5);           % a1
    if( any(ChannelSOS(1:ChannelNumStages,1) == 0 ))
    ChannelCoeffs(3+ts,1) = 0;                 % b2/b0
    ChannelCoeffs(4+ts,1) = 0;                 % b1/b0
    else
    ChannelCoeffs(3+ts,1) = ...
        ChannelSOS(1:ChannelNumStages,3)./ ...
        ChannelSOS(1:ChannelNumStages,1);  % b2/b0
    ChannelCoeffs(4+ts,1) = ...
        ChannelSOS(1:ChannelNumStages,2)./ ...
        ChannelSOS(1:ChannelNumStages,1);  % b1/b0
    end
    
    % length of Cuurent Channel Coeffs
    
    ChannelCoeffsLength = 1+4*ChannelNumStages;
    
    % Offset into coefficient array for the current channel
    offset = (i-1)+4*sum(PoolNumStages(1:i-1));
    
    % Verify that the SOS does not violate the maximum number of stages
    % allocated for the pool
    PoolNumStages(i) = int32(ChannelNumStages);
    if sum(PoolNumStages) > MaxNumStages
        TranslateError('Too many second order sections');
    end

    % Store the coefficients
    PoolCoeffs(offset+(1:ChannelCoeffsLength)) = single(ChannelCoeffs(1:ChannelCoeffsLength));   
end
end

== matlab function TrebleBoost/TrebleBoostStereo/Treble Boost/Ramper/MATLAB Function ==
  data: audioIn input; audioOut output single; targetGain input; rampCoef input
function audioOut = TrebleBoostRamper(audioIn, targetGain, rampCoef)
%#codegen

% input/output
[n,m] = size(audioIn);
audioOut = zeros(n,m, 'single');

persistent previousGain;

% Initialize previousGain
if(isempty(previousGain))
    previousGain = single(1);  
end

targetGain_linear = 10^(targetGain/20);

% Ramp Setup
bRamp = [(1-rampCoef)];
aRamp = [1 -rampCoef];
gain = ones(n,1)*targetGain_linear;

% Ramp Gain
zi = rampCoef*previousGain;     % Initial Conditions
currentGain = filter(bRamp,aRamp,gain,zi);
previousGain = currentGain(end);

currentGain = currentGain*ones(1,m, 'single');

% Apply the gain
audioOut = currentGain.*audioIn;

end

== matlab function TrebleBoost/TrebleBoostStereo/Treble Boost/Ramper/Ramp Coefficient/Trivial Translation ==
  data: rampCoef output; timeConstant input; sampleRate parameter
  events: trigger input FUNCTION_CALL_EVENT
function rampCoef  = fcn(timeConstant, sampleRate)
%#codegen
%[Param:sampleRate]

tau = timeConstant.Value;
Fs = sampleRate;

rampFreq = 1/(2*pi*tau);

rampWc = 2*pi*rampFreq/Fs;
rampSinCoef = sin(rampWc);
rampCosCoef = cos(rampWc);

rampCoef =  (1-rampSinCoef)/rampCosCoef;

end

== matlab function TrebleBoost/TrebleBoostStereo/Compressed Audio Identifier/Boost Decision/Confidence Rate of Decay/Trivial Translation ==
  data: decay output; timeConstant input; sampleRate parameter; fftFrameSize parameter
  events: trigger input FUNCTION_CALL_EVENT
function decay  = fcn(timeConstant, sampleRate, fftFrameSize)
%#codegen
%[Param:sampleRate]
%[Param:fftFrameSize]

tau = timeConstant.Value;
Fd = sampleRate/fftFrameSize;

decay = exp(-1/(tau*Fd));

end

== matlab function TrebleBoost/TrebleBoostStereo/Compressed Audio Identifier/Boost Decision/Hysteresis ==
  data: hysteresisFlag input single; hysteresisFlag output; smoothedConfidence input; confidenceThreshold input; hysteresisBand input
function hysteresisFlag = boostEnable(hysteresisFlag, smoothedConfidence, confidenceThreshold, hysteresisBand)
%#codegen

lowerDecisionThreshold = confidenceThreshold - hysteresisBand/2;
upperDecisionThreshold = confidenceThreshold + hysteresisBand/2;

if((hysteresisFlag == 0) && (smoothedConfidence > upperDecisionThreshold))
    hysteresisFlag = single(1);
elseif((hysteresisFlag == 1) && (smoothedConfidence < lowerDecisionThreshold))
    hysteresisFlag = single(0);
end

== matlab function TrebleBoost/TrebleBoostStereo/Compressed Audio Identifier/Cutoff Frequency Update/Cut-off Frequency Rate of Decay/Trivial Translation ==
  data: decay output; timeConstant input; sampleRate parameter; fftFrameSize parameter
  events: trigger input FUNCTION_CALL_EVENT
function decay  = fcn(timeConstant, sampleRate, fftFrameSize)
%#codegen
%[Param:sampleRate]
%[Param:fftFrameSize]

tau = timeConstant.Value;
Fd = sampleRate/fftFrameSize;

wc = 1/(tau*Fd);
decay = 1 - ((1-sin(wc))/cos(wc));

end

== matlab function TrebleBoost/TrebleBoostStereo/Compressed Audio Identifier/Cutoff Frequency Update/MATLAB Function ==
  data: expectedSmoothingProduct input single; expectedSmoothingProduct output; instantaneousCutoffFrequency input; confidence input; alpha input; expectedConfidence input single; cutoffFrequencyEstimate output; expectedConfidence output
function [expectedSmoothingProduct, cutoffFrequencyEstimate, expectedConfidence] = updateCutoffFrequency(expectedSmoothingProduct, instantaneousCutoffFrequency, confidence, alpha, expectedConfidence)
%#codegen

% Expected Values
expectedSmoothingProduct = (1-alpha)*expectedSmoothingProduct + alpha*confidence*instantaneousCutoffFrequency;
expectedConfidence = (1-alpha)*expectedConfidence + alpha*confidence;

% Current Estimate of Cutoff Frequency
cutoffFrequencyEstimate = expectedSmoothingProduct/(expectedConfidence+eps('single'));   % eps is added to avoid 1/0 operation

end

== matlab function TrebleBoost/TrebleBoostStereo/Compressed Audio Identifier/Gain Derivation/MATLAB Function ==
  data: boostEnable input; boostGain output; cutoffFrequency input; Freq1Hz input; Freq2Hz input; Freq3Hz input; Gain1dB input; Gain2dB input
function boostGain = deriveGain(boostEnable, cutoffFrequency, Freq1Hz, Freq2Hz, Freq3Hz, Gain1dB, Gain2dB)
%#codegen

boostGain = single(0);

if(boostEnable ~= 0)
    if((cutoffFrequency >= Freq1Hz) && (cutoffFrequency < Freq2Hz))
        boostGain = Gain1dB;
    elseif((cutoffFrequency >= Freq2Hz) && (cutoffFrequency < Freq3Hz))
        boostGain = Gain2dB;
    end
end

== matlab function TrebleBoost/TrebleBoostStereo/Compressed Audio Identifier/Instantaneous Cutoff Frequency Calculation/MATLAB Function ==
  data: inputSpectrum input; instantaneousCutoffFrequency output; smoothedSpectrum input; confidence output; minSteepnessThresholddB input; maxSteepnessThresholddB input; minSteepnessValue input; highFrequencyIndex input; energyConfidenceInflectionPoint input; highFrequencyMinEnergyThreshold input; highFrequencyMaxEnergyThreshold input; fullBandFrequencyHz input; minDetectionFrequencyIndex parameter; maxDetectionFrequencyIndex parameter; spectrumSize parameter; frequencies parameter; steepnessIndexRange parameter
function [instantaneousCutoffFrequency, confidence] = Fc_ConfidenceCalc( ...
    inputSpectrum, ...
    smoothedSpectrum, ...
    minSteepnessThresholddB, ...
    maxSteepnessThresholddB, ...
    minSteepnessValue, ...
    highFrequencyIndex, ...
    energyConfidenceInflectionPoint, ...
    highFrequencyMinEnergyThreshold, ...
    highFrequencyMaxEnergyThreshold, ...
    fullBandFrequencyHz, ...
    minDetectionFrequencyIndex, ...
    maxDetectionFrequencyIndex, ...
    spectrumSize, ...
    frequencies, ...
    steepnessIndexRange)
%#codegen
%[Param:minDetectionFrequencyIndex]
%[Param:maxDetectionFrequencyIndex]
%[Param:spectrumSize]
%[Param:frequencies]
%[Param:steepnessIndexRange]

minIndex = minDetectionFrequencyIndex;
maxIndex = maxDetectionFrequencyIndex;

% Initialize confidence and instantaneous cutoff frequency for the loop
confidence = single(0);
instantaneousCutoffFrequency = frequencies(maxIndex);

% Compute dB spectrum
dBSpectrum = 10*log10(max(smoothedSpectrum, eps('single')));

% Calculate the normalized total energy
totalEnergyNorm = sum(smoothedSpectrum)/spectrumSize;

% Loop over the detection range
for k = maxIndex:-1:minIndex
    
    % Calculate Steepness
    topIndex = min(k+steepnessIndexRange,spectrumSize);
    bottomIndex = max(1,k-steepnessIndexRange+1);
    steepness = max(dBSpectrum(bottomIndex:k)) - min(dBSpectrum(k+1:topIndex));
    % Map steepness to a value of [0,1]
    % --- its contribution to the confidence measure
    steepnessConfidence = ((min(max(steepness,minSteepnessThresholddB), maxSteepnessThresholddB) ...
        - minSteepnessThresholddB) * (1-minSteepnessValue) / (maxSteepnessThresholddB - minSteepnessThresholddB) ...
        + (min(steepness,minSteepnessThresholddB)) * minSteepnessValue / minSteepnessThresholddB);
    % Calculate normalized stop-band energy
    stopEnergyNorm = sum(smoothedSpectrum((k+1):end))/single(spectrumSize-k)/totalEnergyNorm;
    % Map stop-band energy to a value of [0,1]
    % --- its contribution to the confidence measure
    energyConfidence = ((1-energyConfidenceInflectionPoint)/energyConfidenceInflectionPoint) ...
        * (energyConfidenceInflectionPoint - min(stopEnergyNorm, energyConfidenceInflectionPoint)) ...
        + (energyConfidenceInflectionPoint /(1-energyConfidenceInflectionPoint)) ...
        * (1 - max(stopEnergyNorm, energyConfidenceInflectionPoint));
    % Candidate for the highest confidence measure
    confidenceCandidate = steepnessConfidence * energyConfidence ;
    % Replace if necessary
    if confidenceCandidate > confidence
        confidence = confidenceCandidate;
        instantaneousCutoffFrequency = frequencies(k);
    end
    
end

%% Confidence Cutoff Frequency Calculation Special
% Calculate energy in the high frequencies
highFrequencyEnergy = sum(inputSpectrum(highFrequencyIndex+1:spectrumSize));

% Map high-frequency energy to a value of [0,1]
% --- Candidate for the confidence measure
confidenceCandidate = min(1,max(0,(highFrequencyEnergy - highFrequencyMinEnergyThreshold)/ ...
    (highFrequencyMaxEnergyThreshold - highFrequencyMinEnergyThreshold)));

% Replace if necessary
if confidenceCandidate > confidence
    instantaneousCutoffFrequency = fullBandFrequencyHz;
    confidence = confidenceCandidate;
end

end
